simulink model "Lab5"  (R2022b)
settings: Solver=VariableStepAuto  StartTime=0.0  StopTime=t_simulation  RelTol=1e-3
values from neighbouring files (symbols this model uses):
  dgq = 0.1*qgN    (= 1000)    [porownani.m]
  dTzew = 0    [porownani.m]
  L11 = [ Cvp (Kcwp + Kcp)]    [porownani.m]
  L12 = [ (Cvp*Kcw) (Kcw*Kcwp + Kcp*Kcw + Kcwp*Kcp)]    [porownani.m]
  L21 = Kcwp    (= 58.8235294118)    [porownani.m]
  L22 = [ (Cvw*Kcp)  (Kcw*Kcp + Kcp*Kcwp + Kcwp*Kcw)]    [porownani.m]
  M = [(Cvw*Cvp) (Kcwp*Cvw + Kcp*Cvw + Kcw*Cvp + Kcwp*Cvp) (Kcw*Kcwp + Kcw*Kcp + Kcp*Kcwp)]    [porownani.m]
  t0 = 500    [porownani.m]
  Tp0 = (Kcp*Tzew0 + Kcwp * Twew0)/(Kcwp + Kcp)    (= 3)    [porownani.m]
  Twew0 = ((qg0*(Kcp + Kcwp))/(Kcwp*Kcw + Kcp * Kcw + Kcp * Kcwp)) + Tzew0    (= 9)    [porownani.m]
settings Model: Creator=huber  LastModifiedBy=huber
settings DataIOCC: ReturnWorkspaceOutputs=off

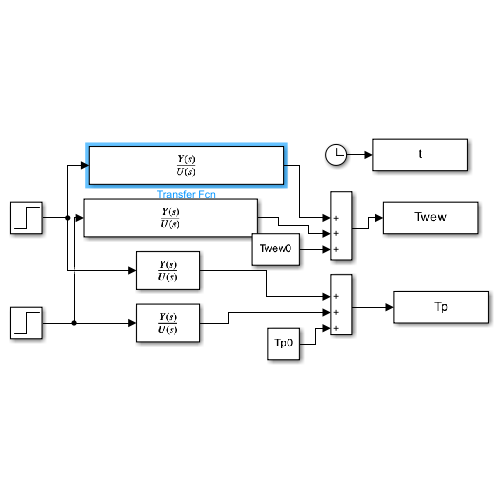
[thumbnail: Simulink's stored preview of the top-level diagram]
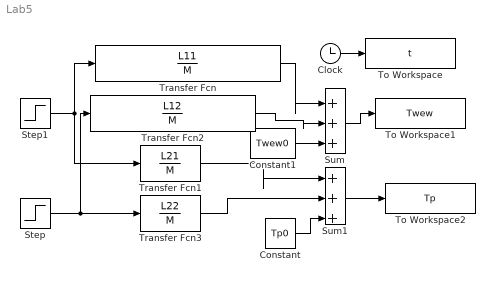
== system Lab5 ==
  Clock : Clock
  Constant : Constant  Value=Tp0
  Constant1 : Constant  Value=Twew0
  Step : Step  Time=t0  After=dTzew  SampleTime=0
  Step1 : Step  Time=t0  After=dgq  SampleTime=0
  Sum : Sum  Inputs=|+++
  Sum1 : Sum  Inputs=|+++
  To Workspace : ToWorkspace  VariableName=t  SampleTime=-1
  To Workspace1 : ToWorkspace  VariableName=Twew  SampleTime=-1
  To Workspace2 : ToWorkspace  VariableName=Tp  SampleTime=-1
  Transfer Fcn : TransferFcn  Numerator=L11  Denominator=M
  Transfer Fcn1 : TransferFcn  Numerator=L21  Denominator=M
  Transfer Fcn2 : TransferFcn  Numerator=L12  Denominator=M
  Transfer Fcn3 : TransferFcn  Numerator=L22  Denominator=M
  wires:
  Clock/1 -> To Workspace/1
  Step/1 -> Transfer Fcn3/1, Transfer Fcn2/1
  Step1/1 -> Transfer Fcn1/1, Transfer Fcn/1
  Transfer Fcn/1 -> Sum/1
  Transfer Fcn2/1 -> Sum/2
  Transfer Fcn1/1 -> Sum1/1
  Transfer Fcn3/1 -> Sum1/2
  Sum1/1 -> To Workspace2/1
  Sum/1 -> To Workspace1/1
  Constant/1 -> Sum1/3
  Constant1/1 -> Sum/3
